simulink model "ACtoDC_WPT_current"  (R2018a)
settings: Solver=FixedStepAuto  StartTime=0.0  StopTime=stopTime  FixedStep=sampleTime  RelTol=1e-3
InitFcn:
  | fs=150e3; %Hz
  | wo=2*pi*fs;
  | stopTime=0.1;
  | sampleTime=1e-8;
  | deadtime= round(((1/fs)/20)/sampleTime);
  | Vdc=100;
  | Lp=82e-6;
  | Ls=66e-6;
  | Cs=1/ (Ls*4*pi*pi*150e3*150e3);
  | Rp=0.3;
  | Rs=0.2;
  | RLOAD=40
  | k=0.2;
  | M=sqrt(Lp*Ls)*k;
  | Cout=1e-6; %F
  | Cp=Lp/((wo^4*M^4/RLOAD)+(wo^2*Lp^2))
libraries: powerlib x18
settings Model: Creator=enes_  LastModifiedBy=enes_

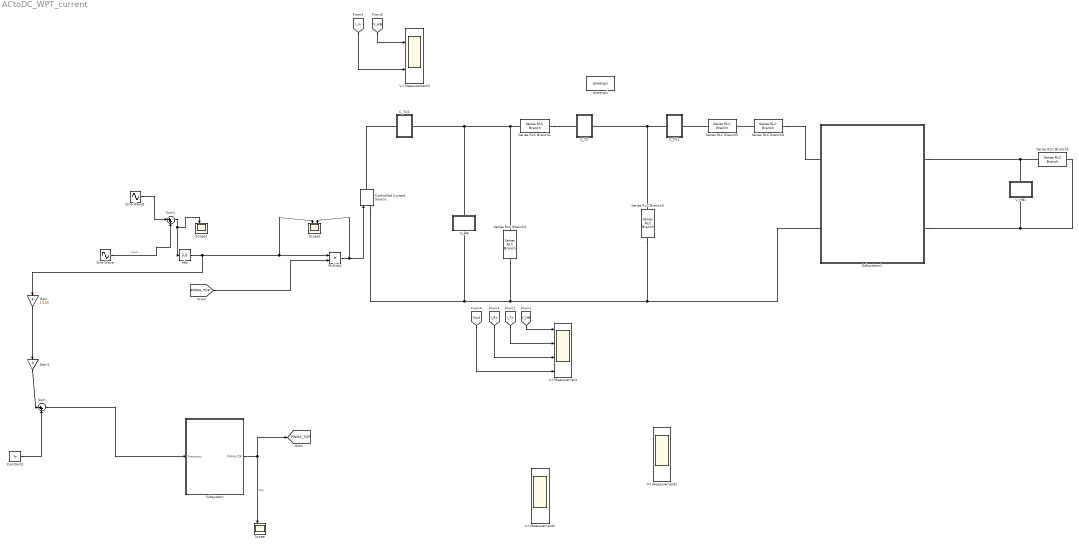
== system ACtoDC_WPT_current ==
  Abs : Abs
  C_TX : Subsystem
  C_TX1 : Subsystem
  C_TX2 : Subsystem
  Constant2 : Constant  Value=fs
  Controlled Current Source : powerlib/Electrical Sources/Controlled Current Source  Initialize=on  Source_Type=AC  Amplitude=0  Phase=0  Frequency=0  Measurements=None
  Gain : Gain  Gain=1/100
  Gain1 : Gain  Gain=0
  Multiply : Product
  Scope : Scope  NumInputPorts=2
  Scope1 : Scope  NumInputPorts=2
  Scope2 : Scope  NumInputPorts=2
  Series RLC Branch1 : powerlib/Elements/Series RLC Branch  LConnTagsString=__new0  RConnTagsString=__new0  BranchType=R  Resistance=RLOAD  Inductance=Lp  SetiL0=off  InitialCurrent=0  Capacitance=Cp  Setx0=off  InitialVoltage=0  Measurements=None
  Series RLC Branch2 : powerlib/Elements/Series RLC Branch  LConnTagsString=__new0  RConnTagsString=__new0  BranchType=L  Resistance=Rp  Inductance=Lp-M  SetiL0=off  InitialCurrent=0  Capacitance=Cp  Setx0=off  InitialVoltage=0  Measurements=None
  Series RLC Branch3 : powerlib/Elements/Series RLC Branch  LConnTagsString=__new0  RConnTagsString=__new0  BranchType=L  Resistance=Rp  Inductance=M  SetiL0=off  InitialCurrent=0  Capacitance=Cp  Setx0=off  InitialVoltage=0  Measurements=None
  Series RLC Branch4 : powerlib/Elements/Series RLC Branch  LConnTagsString=__new0  RConnTagsString=__new0  BranchType=C  Resistance=Rp  Inductance=Lp  SetiL0=off  InitialCurrent=0  Capacitance=Cp  Setx0=off  InitialVoltage=0  Measurements=None
  Series RLC Branch5 : powerlib/Elements/Series RLC Branch  LConnTagsString=__new0  RConnTagsString=__new0  BranchType=L  Resistance=Rp  Inductance=Ls-M  SetiL0=off  InitialCurrent=0  Capacitance=Cp  Setx0=off  InitialVoltage=0  Measurements=None
  Series RLC Branch6 : powerlib/Elements/Series RLC Branch  LConnTagsString=__new0  RConnTagsString=__new0  BranchType=C  Resistance=Rp  Inductance=Lp  SetiL0=off  InitialCurrent=0  Capacitance=Cs  Setx0=off  InitialVoltage=0  Measurements=None
  Sine Wave : Sin  Amplitude=5  Frequency=2*pi*50  SampleTime=0
  Sine Wave1 : Sin  Amplitude=0  Frequency=2*pi*50*3  SampleTime=0
  Subsystem : Subsystem
  Subsystem1 : Subsystem
  Sum : Sum  Inputs=|++
  Sum1 : Sum  Inputs=|++
  V-I Measurement : Scope  NumInputPorts=4
  V-I Measurement1 : Scope  NumInputPorts=4
  V-I Measurement2 : Scope  NumInputPorts=2
  V-I Measurement3 : Scope  NumInputPorts=2
  V_HB : Subsystem
  V_HB1 : Subsystem
  powergui : powerlib/powergui  Priority=1  SimulationMode=Discrete  SampleTime=sampleTime  frequency=60  Iterations=50  frequencyindice=0  Pbase=100e6  ErrMax=1e-4  UnitsV=kV  UnitsW=MW  buscounter=0  FunctionMessages=off  echomessages=off  EnableUseOfTLC=off  CurrentSourceSwitches=off  DisableSnubberDevices=off  DisableRonSwitches=off  DisableVfSwitches=off  DisplayEquations=off  SolverType=Tustin/Backward Euler (TBE)  Interpol=off  ExternalGateDelay=off  methode=off  Ts=100  x0status=blocks  SPID=off  SwTol=0  HookPort=off  RestoreLinks=warning  ResistiveCurrentMeasurement=off  Frange=[0:2:500]  Ylog=off  Xlog=on  ShowGrid=off  save=off  variable=ZData  structure=ScopeData2  ZoomFFT=off  StartTime=0.0  cycles=4  DisplayStyle=2  fundamental=100  FreqAxis=off  MaxFrequency=600e3  frequencyindicesteady=1  RmsSteady=1  display=off
  tag scope: PWMA_TOP=global
  wires:
  Subsystem/1(PWMA_TOP) -> [PWMA_TOP], Scope/1  "TA+"
  Sine Wave/1 -> Sum1/2  "Input"
  Abs/1 -> Gain/1, Scope1/1, Multiply/1
  [PWMA_TOP] -> Multiply/2
  Multiply/1 -> Controlled Current Source/1, Scope1/2
  [V_HB] -> V-I Measurement/1
  [I_Tx] -> V-I Measurement/2
  [I_Rx] -> V-I Measurement/3
  [Vout] -> V-I Measurement/4
  Constant2/1 -> Sum/2
  Sum/1 -> Subsystem/1(Frequency)
  Gain/1 -> Gain1/1
  Sine Wave1/1 -> Sum1/1
  Sum1/1 -> Scope2/1, Abs/1
  Gain1/1 -> Sum/1
  [V_HB] -> V-I Measurement3/1
  [I_in] -> V-I Measurement3/2
  connections:
  Subsystem1/RConn2 -- V_HB1/LConn1 -- Series RLC Branch1/LConn1
  Series RLC Branch3/RConn1 -- Subsystem1/LConn2 -- Series RLC Branch4/RConn1 -- Controlled Current Source/LConn1 -- V_HB/LConn1
  Series RLC Branch5/LConn1 -- C_TX1/RConn1
  Series RLC Branch2/RConn1 -- C_TX/LConn1
  V_HB/RConn1 -- Series RLC Branch2/LConn1 -- Series RLC Branch4/LConn1 -- C_TX2/LConn1
  Series RLC Branch6/LConn1 -- Series RLC Branch5/RConn1
  Series RLC Branch6/RConn1 -- Subsystem1/LConn1
  Series RLC Branch3/LConn1 -- C_TX1/LConn1 -- C_TX/RConn1
  Series RLC Branch1/RConn1 -- Subsystem1/RConn1 -- V_HB1/RConn1
  C_TX2/RConn1 -- Controlled Current Source/RConn1

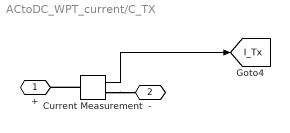
== system ACtoDC_WPT_current/C_TX ==
  Current Measurement : powerlib/Measurements/Current Measurement  PhasorSimulation=off  OutputType=Complex  PSBequivalent=0
  + : PMIOPort  Side=Left
  - : PMIOPort  Port=2  Side=Right
  tag scope: I_Tx=global
  wires:
  Current Measurement/1 -> [I_Tx]
  connections:
  Current Measurement/RConn1 -- -/RConn1
  Current Measurement/LConn1 -- +/RConn1

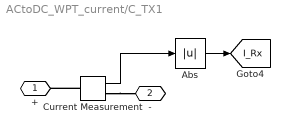
== system ACtoDC_WPT_current/C_TX1 ==
  Abs : Abs
  Current Measurement : powerlib/Measurements/Current Measurement  PhasorSimulation=off  OutputType=Complex  PSBequivalent=0
  + : PMIOPort  Side=Left
  - : PMIOPort  Port=2  Side=Right
  tag scope: I_Rx=global
  wires:
  Current Measurement/1 -> Abs/1
  Abs/1 -> [I_Rx]
  connections:
  Current Measurement/RConn1 -- -/RConn1
  Current Measurement/LConn1 -- +/RConn1

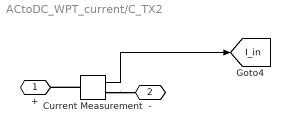
== system ACtoDC_WPT_current/C_TX2 ==
  Current Measurement : powerlib/Measurements/Current Measurement  PhasorSimulation=off  OutputType=Complex  PSBequivalent=0
  + : PMIOPort  Side=Left
  - : PMIOPort  Port=2  Side=Right
  tag scope: I_in=global
  wires:
  Current Measurement/1 -> [I_in]
  connections:
  Current Measurement/RConn1 -- -/RConn1
  Current Measurement/LConn1 -- +/RConn1

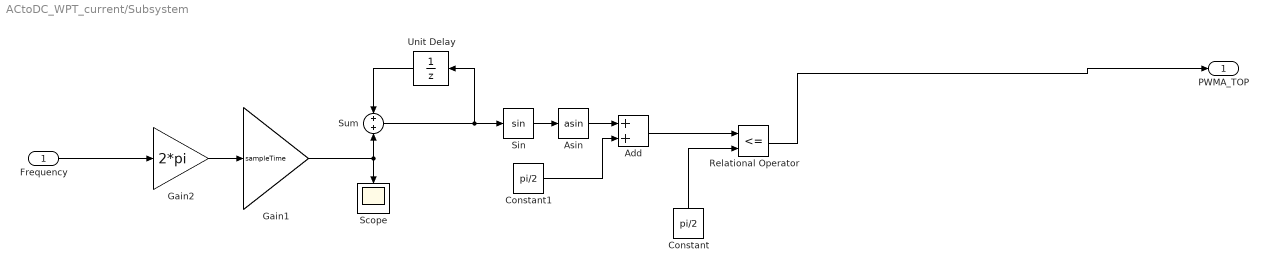
== system ACtoDC_WPT_current/Subsystem ==
  Frequency : Inport
  Add : Sum
  Asin : Trigonometry  Operator=asin
  Constant : Constant  Value=pi/2
  Constant1 : Constant  Value=pi/2
  Gain1 : Gain  Gain=sampleTime
  Gain2 : Gain  Gain=2*pi
  Relational Operator : RelationalOperator  Operator=<=  OutDataTypeStr=boolean  RndMeth=Simplest
  Scope : Scope
  Sin : Trigonometry
  Sum : Sum
  Unit Delay : UnitDelay  SampleTime=-1
  PWMA_TOP : Outport
  wires:
  Gain1/1 -> Sum/2, Scope/1
  Relational Operator/1 -> PWMA_TOP/1
  Asin/1 -> Add/1
  Sum/1 -> Sin/1, Unit Delay/1
  Gain2/1 -> Gain1/1
  Unit Delay/1 -> Sum/1
  Frequency/1 -> Gain2/1
  Add/1 -> Relational Operator/1
  Sin/1 -> Asin/1
  Constant1/1 -> Add/2
  Constant/1 -> Relational Operator/2

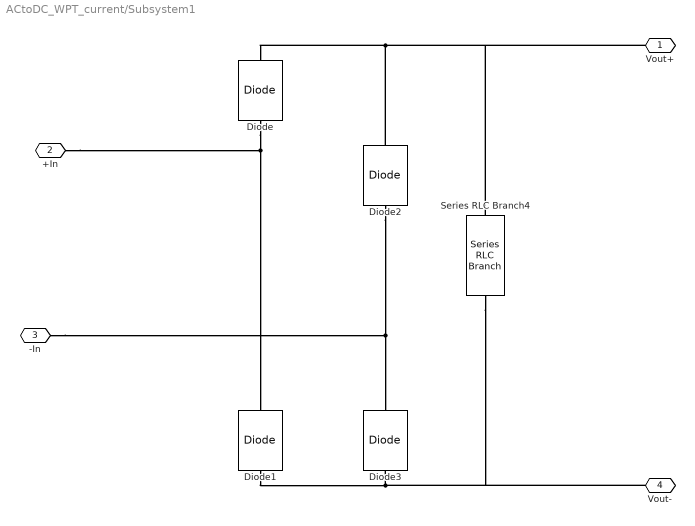
== system ACtoDC_WPT_current/Subsystem1 ==
  Diode{,1..3} (4 alike) : powerlib/Power Electronics/Diode  Ron=0.001  Lon=0  Vf=0.8  IC=0  UseSnubber=0  Rs=500  Cs=250e-9  Measurements=off
  Series RLC Branch4 : powerlib/Elements/Series RLC Branch  LConnTagsString=__new0  RConnTagsString=__new0  BranchType=C  Resistance=RLOAD  Inductance=Lp  SetiL0=off  InitialCurrent=0  Capacitance=Cout  Setx0=off  InitialVoltage=0  Measurements=None
  Vout+ : PMIOPort  Side=Right
  +In : PMIOPort  Port=2  Side=Left
  -In : PMIOPort  Port=3  Side=Left
  Vout- : PMIOPort  Port=4  Side=Right
  connections:
  Diode/LConn1 -- +In/RConn1 -- Diode1/RConn1
  Vout+/RConn1 -- Series RLC Branch4/LConn1 -- Diode/RConn1 -- Diode2/RConn1
  -In/RConn1 -- Diode3/RConn1 -- Diode2/LConn1
  Vout-/RConn1 -- Series RLC Branch4/RConn1 -- Diode1/LConn1 -- Diode3/LConn1

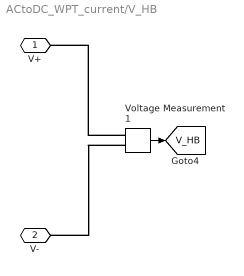
== system ACtoDC_WPT_current/V_HB ==
  Voltage Measurement1 : powerlib/Measurements/Voltage Measurement  PhasorSimulation=off  OutputType=Complex  PSBequivalent=0
  V+ : PMIOPort  Side=Right
  V- : PMIOPort  Port=2  Side=Left
  tag scope: V_HB=global
  wires:
  Voltage Measurement1/1 -> [V_HB]
  connections:
  Voltage Measurement1/LConn1 -- V+/RConn1
  Voltage Measurement1/LConn2 -- V-/RConn1

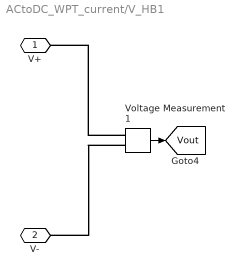
== system ACtoDC_WPT_current/V_HB1 ==
  Voltage Measurement1 : powerlib/Measurements/Voltage Measurement  PhasorSimulation=off  OutputType=Complex  PSBequivalent=0
  V+ : PMIOPort  Side=Right
  V- : PMIOPort  Port=2  Side=Left
  tag scope: Vout=global
  wires:
  Voltage Measurement1/1 -> [Vout]
  connections:
  Voltage Measurement1/LConn1 -- V+/RConn1
  Voltage Measurement1/LConn2 -- V-/RConn1
